simulink model "q2b"  (R2024a)
settings: Solver=VariableStepAuto  StartTime=0.0  StopTime=10  MaxStep=1e-4  RelTol=1e-3
settings Model: Creator=SHINE MOHAN S  LastModifiedBy=SHINE MOHAN S

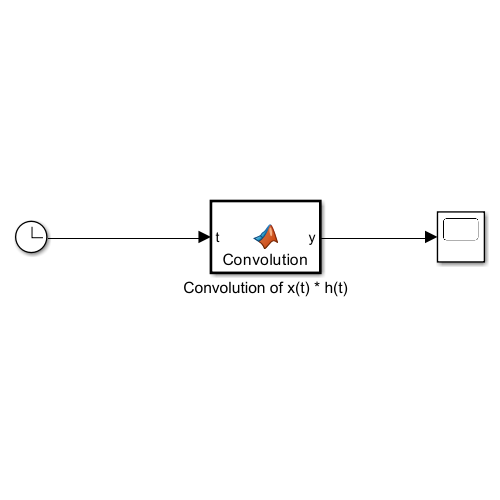
[thumbnail: Simulink's stored preview of the top-level diagram]
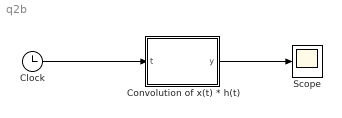
== system q2b ==
  Clock : Clock
  Convolution of x(t) * h(t) : MATLAB Function  TreatAsAtomicUnit=on
  Scope : Scope
  wires:
  Clock/1 -> Convolution of x(t) * h(t)/1(t)
  Convolution of x(t) * h(t)/1(y) -> Scope/1

== matlab function q2b/Convolution of x(t) * h(t) ==
  data: t input; y output
function y = Convolution(t)
    % Define x(t) function
    function x_val = x_func(tau)
        if tau >= 0 && tau < 3
            x_val = 1;
        else
            x_val = 0;
        end
    end

    % Define h(t) function
    function h_val = h_func(tau)
        if tau >= 0
            h_val = exp(-tau);
        else
            h_val = 0;
        end
    end

    % Adjust tau for more accurate approximation
    tau = linspace(0, t, 5000); % Finer sampling, limited range based on support of x and h
    dt = tau(2) - tau(1);
    
    % Initialize output
    y = 0;

    % Calculate convolution
    for i = 1:length(tau)
        t_tau = t - tau(i);
        x_tau = x_func(tau(i));
        h_tau = h_func(t_tau);
        y = y + x_tau * h_tau * dt; % Multiply by dt for approximation
    end
end
